simulink model "paliotta"  (Simulink 7.9)
settings: Solver=ode3  StartTime=0.0  StopTime=1000  FixedStep=0.05  RelTol=1e-3
libraries: simulink x3
settings Model: Creator=Staciej  LastModifiedBy=Staciej  CovModelRefEnable=off
settings DataIOCC: LimitDataPoints=off  SaveFormat=StructureWithTime  SignalLoggingSaveFormat=Dataset
settings OptimizationCC: ExpressionDepthLimit=128
settings DebuggingCC: UnderspecifiedInitializationDetection=Simplified  MergeDetectMultiDrivingBlocksExec=error  SolverPrmCheckMsg=none  FrameProcessingCompatibilityMsg=error  StateNameClashWarn=none
settings HardwareCC: ProdBitPerPointer=64  ProdLargestAtomicFloat=Float  ProdIntDivRoundTo=Zero  ProdEndianess=LittleEndian  ProdHWDeviceType=Specified
settings ModelReferenceCC: PropagateSignalLabelsOutOfModel=on
settings CodeAppCC: CustomSymbolStrType=$N$R$M_T
settings GRTTargetCC: CodeReplacementLibrary=C89/C90 (ANSI)

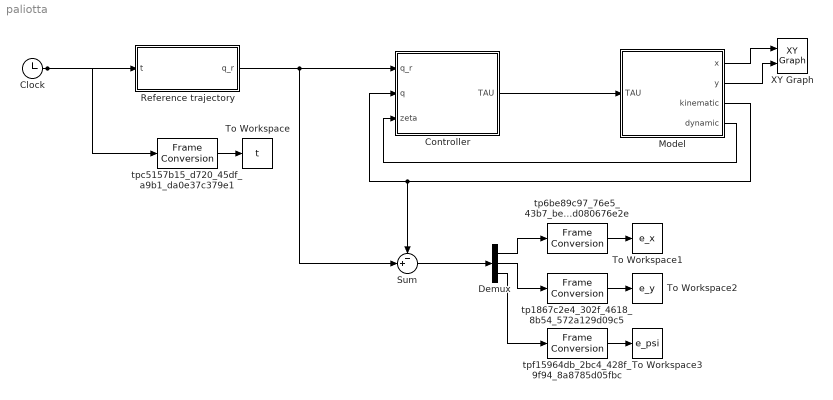
== system paliotta ==
  Clock : Clock
  Controller : Subsystem
  Demux : Demux  Outputs=3
  Model : Subsystem
  Reference trajectory : Subsystem
  Sum : Sum  Inputs=-+|
  To Workspace : ToWorkspace  VariableName=t  SampleTime=-1
  To Workspace1 : ToWorkspace  VariableName=e_x  SampleTime=-1
  To Workspace2 : ToWorkspace  VariableName=e_y  SampleTime=-1
  To Workspace3 : ToWorkspace  VariableName=e_psi  SampleTime=-1
  XY Graph : simulink/Sinks/XY Graph  xmin=-100  xmax=1000  ymin=-200  ymax=200  st=-1
  tp1867c2e4_302f_4618_8b54_572a129d09c5 : FrameConversion  InheritSamplingMode=off  OutFrame=Sample-based
  tp6be89c97_76e5_43b7_be9f_a8d080676e2e : FrameConversion  InheritSamplingMode=off  OutFrame=Sample-based
  tpc5157b15_d720_45df_a9b1_da0e37c379e1 : FrameConversion  InheritSamplingMode=off  OutFrame=Sample-based
  tpf15964db_2bc4_428f_9f94_8a8785d05fbc : FrameConversion  InheritSamplingMode=off  OutFrame=Sample-based
  wires:
  Clock/1 -> Reference trajectory/1(t), tpc5157b15_d720_45df_a9b1_da0e37c379e1/1
  Model/1(x) -> XY Graph/1
  Model/2(y) -> XY Graph/2
  Reference trajectory/1(q_r) -> Controller/1(q_r), Sum/2
  Model/4(dynamic) -> Controller/3(zeta)
  Model/3(kinematic) -> Controller/2(q), Sum/1
  Sum/1 -> Demux/1
  Controller/1(TAU) -> Model/1(TAU)
  tpc5157b15_d720_45df_a9b1_da0e37c379e1/1 -> To Workspace/1
  Demux/1 -> tp6be89c97_76e5_43b7_be9f_a8d080676e2e/1
  tp6be89c97_76e5_43b7_be9f_a8d080676e2e/1 -> To Workspace1/1
  Demux/2 -> tp1867c2e4_302f_4618_8b54_572a129d09c5/1
  tp1867c2e4_302f_4618_8b54_572a129d09c5/1 -> To Workspace2/1
  Demux/3 -> tpf15964db_2bc4_428f_9f94_8a8785d05fbc/1
  tpf15964db_2bc4_428f_9f94_8a8785d05fbc/1 -> To Workspace3/1

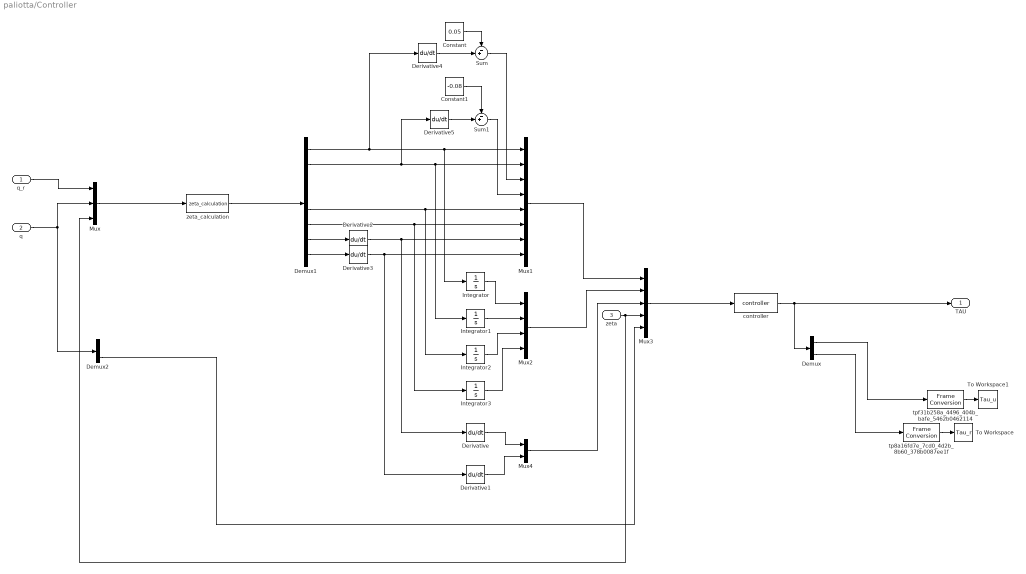
== system paliotta/Controller ==
  q_r : Inport
  q : Inport  Port=2
  zeta : Inport  Port=3
  Constant : Constant  Value=0.05
  Constant1 : Constant  Value=-0.08
  Demux : Demux  Outputs=2
  Demux1 : Demux  Outputs=8
  Demux2 : Demux  Outputs=3
  Derivative{,1..5} (6 alike) : Derivative
  Integrator{,1..3} (4 alike) : Integrator
  Mux : Mux  Inputs=3
  Mux1 : Mux  Inputs=8
  Mux2 : Mux
  Mux3 : Mux  Inputs=5
  Mux4 : Mux  Inputs=2
  Sum : Sum  Inputs=-+|
  Sum1 : Sum  Inputs=-+|
  To Workspace : ToWorkspace  VariableName=Tau_r  SampleTime=-1
  To Workspace1 : ToWorkspace  VariableName=Tau_u  SampleTime=-1
  controller : MATLABFcn  MATLABFcn=controller  OutputDimensions=2
  tp8a16fd7e_7cd0_4d2b_8b60_378b0087ee1f : FrameConversion  InheritSamplingMode=off  OutFrame=Sample-based
  tpf31b258a_4496_404b_bafe_5462b0462114 : FrameConversion  InheritSamplingMode=off  OutFrame=Sample-based
  zeta_calculation : MATLABFcn  MATLABFcn=zeta_calculation  OutputDimensions=8
  TAU : Outport
  wires:
  controller/1 -> TAU/1, Demux/1
  q_r/1 -> Mux/1
  q/1 -> Demux2/1, Mux/2
  Mux/1 -> zeta_calculation/1
  zeta_calculation/1 -> Demux1/1
  Demux1/1 -> Derivative4/1, Integrator/1, Mux1/1
  Demux1/2 -> Derivative5/1, Integrator1/1, Mux1/2
  Demux1/5 -> Integrator2/1, Mux1/5
  Demux1/6 -> Integrator3/1, Mux1/6
  Demux1/7 -> Derivative2/1
  Demux1/8 -> Derivative3/1
  Integrator/1 -> Mux2/1
  Integrator1/1 -> Mux2/2
  Integrator2/1 -> Mux2/3
  Integrator3/1 -> Mux2/4
  Mux1/1 -> Mux3/1
  Mux2/1 -> Mux3/2
  Mux3/1 -> controller/1
  zeta/1 -> Mux/3, Mux3/4
  Demux2/3 -> Mux3/5
  Derivative1/1 -> Mux4/2
  Derivative/1 -> Mux4/1
  Mux4/1 -> Mux3/3
  Derivative2/1 -> Derivative/1, Mux1/7
  Derivative3/1 -> Derivative1/1, Mux1/8
  Constant/1 -> Sum/1
  Derivative4/1 -> Sum/2
  Derivative5/1 -> Sum1/2
  Constant1/1 -> Sum1/1
  Sum/1 -> Mux1/3
  Sum1/1 -> Mux1/4
  Demux/2 -> tp8a16fd7e_7cd0_4d2b_8b60_378b0087ee1f/1
  tp8a16fd7e_7cd0_4d2b_8b60_378b0087ee1f/1 -> To Workspace/1
  Demux/1 -> tpf31b258a_4496_404b_bafe_5462b0462114/1
  tpf31b258a_4496_404b_bafe_5462b0462114/1 -> To Workspace1/1

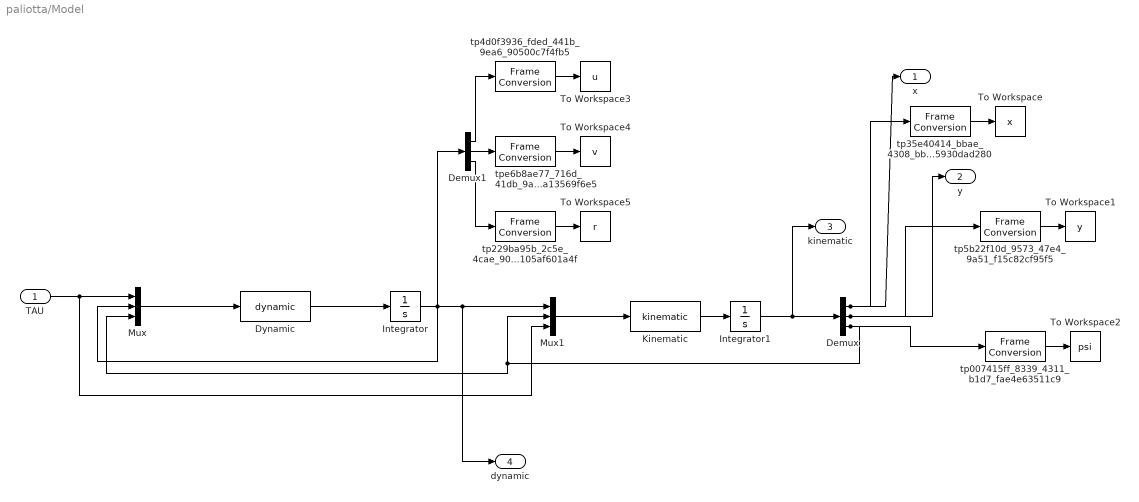
== system paliotta/Model ==
  TAU : Inport
  Demux : Demux  Outputs=3
  Demux1 : Demux  Outputs=3
  Dynamic : MATLABFcn  MATLABFcn=dynamic  OutputDimensions=3
  Integrator : Integrator  InitialCondition=[0 0 0]
  Integrator1 : Integrator  InitialCondition=[5 10 0]
  Kinematic : MATLABFcn  MATLABFcn=kinematic  OutputDimensions=3
  Mux : Mux  Inputs=3
  Mux1 : Mux  Inputs=3
  To Workspace : ToWorkspace  VariableName=x  SampleTime=-1
  To Workspace1 : ToWorkspace  VariableName=y  SampleTime=-1
  To Workspace2 : ToWorkspace  VariableName=psi  SampleTime=-1
  To Workspace3 : ToWorkspace  VariableName=u  SampleTime=-1
  To Workspace4 : ToWorkspace  VariableName=v  SampleTime=-1
  To Workspace5 : ToWorkspace  VariableName=r  SampleTime=-1
  tp007415ff_8339_4311_b1d7_fae4e63511c9 : FrameConversion  InheritSamplingMode=off  OutFrame=Sample-based
  tp229ba95b_2c5e_4cae_90d9_8105af601a4f : FrameConversion  InheritSamplingMode=off  OutFrame=Sample-based
  tp35e40414_bbae_4308_bb87_aa5930dad280 : FrameConversion  InheritSamplingMode=off  OutFrame=Sample-based
  tp4d0f3936_fded_441b_9ea6_90500c7f4fb5 : FrameConversion  InheritSamplingMode=off  OutFrame=Sample-based
  tp5b22f10d_9573_47e4_9a51_f15c82cf95f5 : FrameConversion  InheritSamplingMode=off  OutFrame=Sample-based
  tpe6b8ae77_716d_41db_9a37_b8a13569f6e5 : FrameConversion  InheritSamplingMode=off  OutFrame=Sample-based
  x : Outport
  y : Outport  Port=2
  kinematic : Outport  Port=3
  dynamic : Outport  Port=4
  wires:
  TAU/1 -> Mux1/3, Mux/1
  Mux/1 -> Dynamic/1
  Dynamic/1 -> Integrator/1
  Integrator/1 -> Mux/2, Demux1/1, dynamic/1, Mux1/1
  Mux1/1 -> Kinematic/1
  Kinematic/1 -> Integrator1/1
  Demux/3 -> Mux/3, Mux1/2, tp007415ff_8339_4311_b1d7_fae4e63511c9/1
  Demux/1 -> x/1, tp35e40414_bbae_4308_bb87_aa5930dad280/1
  Demux/2 -> y/1, tp5b22f10d_9573_47e4_9a51_f15c82cf95f5/1
  Integrator1/1 -> kinematic/1, Demux/1
  tp35e40414_bbae_4308_bb87_aa5930dad280/1 -> To Workspace/1
  tp5b22f10d_9573_47e4_9a51_f15c82cf95f5/1 -> To Workspace1/1
  tp007415ff_8339_4311_b1d7_fae4e63511c9/1 -> To Workspace2/1
  Demux1/1 -> tp4d0f3936_fded_441b_9ea6_90500c7f4fb5/1
  tp4d0f3936_fded_441b_9ea6_90500c7f4fb5/1 -> To Workspace3/1
  Demux1/2 -> tpe6b8ae77_716d_41db_9a37_b8a13569f6e5/1
  tpe6b8ae77_716d_41db_9a37_b8a13569f6e5/1 -> To Workspace4/1
  Demux1/3 -> tp229ba95b_2c5e_4cae_90d9_8105af601a4f/1
  tp229ba95b_2c5e_4cae_90d9_8105af601a4f/1 -> To Workspace5/1

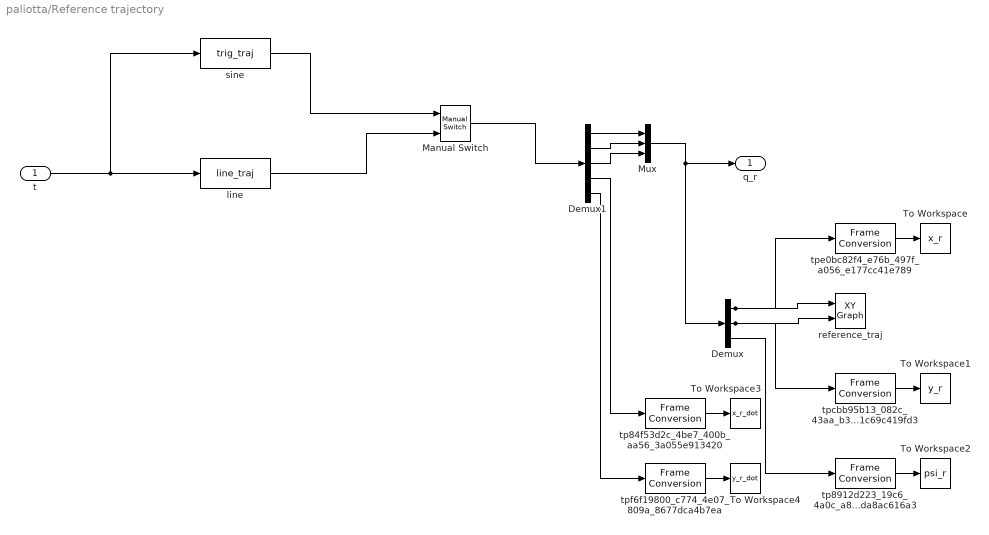
== system paliotta/Reference trajectory ==
  t : Inport
  Demux : Demux  Outputs=3
  Demux1 : Demux  Outputs=5
  Manual Switch : simulink/Signal Routing/Manual Switch  sw=1  action=0  varsize=off
  Mux : Mux  Inputs=3
  To Workspace : ToWorkspace  VariableName=x_r  SampleTime=-1
  To Workspace1 : ToWorkspace  VariableName=y_r  SampleTime=-1
  To Workspace2 : ToWorkspace  VariableName=psi_r  SampleTime=-1
  To Workspace3 : ToWorkspace  VariableName=x_r_dot  SampleTime=-1
  To Workspace4 : ToWorkspace  VariableName=y_r_dot  SampleTime=-1
  line : MATLABFcn  MATLABFcn=line_traj  OutputDimensions=5
  reference_traj : simulink/Sinks/XY Graph  xmin=-100  xmax=1000  ymin=-200  ymax=200  st=-1
  sine : MATLABFcn  MATLABFcn=trig_traj  OutputDimensions=5
  tp84f53d2c_4be7_400b_aa56_3a055e913420 : FrameConversion  InheritSamplingMode=off  OutFrame=Sample-based
  tp8912d223_19c6_4a0c_a8b2_14da8ac616a3 : FrameConversion  InheritSamplingMode=off  OutFrame=Sample-based
  tpcbb95b13_082c_43aa_b3f6_a1c69c419fd3 : FrameConversion  InheritSamplingMode=off  OutFrame=Sample-based
  tpe0bc82f4_e76b_497f_a056_e177cc41e789 : FrameConversion  InheritSamplingMode=off  OutFrame=Sample-based
  tpf6f19800_c774_4e07_809a_8677dca4b7ea : FrameConversion  InheritSamplingMode=off  OutFrame=Sample-based
  q_r : Outport
  wires:
  t/1 -> sine/1, line/1
  Demux/1 -> reference_traj/1, tpe0bc82f4_e76b_497f_a056_e177cc41e789/1
  Demux/2 -> reference_traj/2, tpcbb95b13_082c_43aa_b3f6_a1c69c419fd3/1
  line/1 -> Manual Switch/2
  sine/1 -> Manual Switch/1
  Manual Switch/1 -> Demux1/1
  Demux1/1 -> Mux/1
  Demux1/2 -> Mux/2
  Demux1/3 -> Mux/3
  Mux/1 -> Demux/1, q_r/1
  tpe0bc82f4_e76b_497f_a056_e177cc41e789/1 -> To Workspace/1
  tpcbb95b13_082c_43aa_b3f6_a1c69c419fd3/1 -> To Workspace1/1
  Demux/3 -> tp8912d223_19c6_4a0c_a8b2_14da8ac616a3/1
  tp8912d223_19c6_4a0c_a8b2_14da8ac616a3/1 -> To Workspace2/1
  Demux1/4 -> tp84f53d2c_4be7_400b_aa56_3a055e913420/1
  tp84f53d2c_4be7_400b_aa56_3a055e913420/1 -> To Workspace3/1
  Demux1/5 -> tpf6f19800_c774_4e07_809a_8677dca4b7ea/1
  tpf6f19800_c774_4e07_809a_8677dca4b7ea/1 -> To Workspace4/1
